simulink model "halate_koli"  (R2015a)
settings: Solver=ode45  StartTime=0.02  StopTime=0.04  RelTol=1e-3
libraries: powerlib x41, simulink x14, powerlib_meascontrol x14, dspstat3 x2
settings Model: Creator=yahya  LastModifiedBy=Yahya

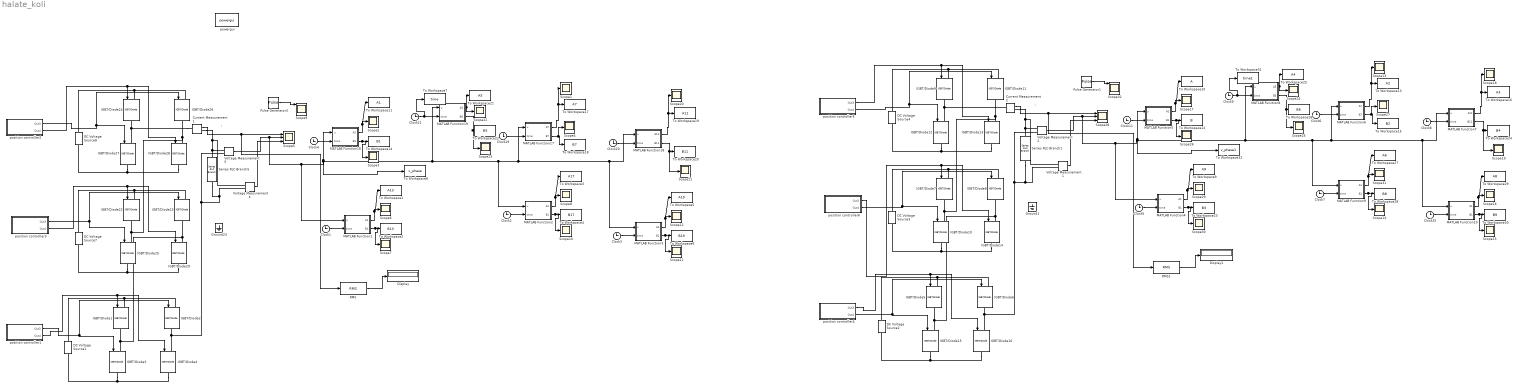
== system halate_koli ==
  note: i
  note: i
  Clock{1..11,19..21} (14 alike) : Clock
  Current Measurement1 : powerlib/Measurements/Current Measurement  PhasorSimulation=off  OutputType=Complex  PSBequivalent=0
  Current Measurement2 : powerlib/Measurements/Current Measurement  PhasorSimulation=off  OutputType=Complex  PSBequivalent=0
  DC Voltage Source{1..4,7..8} (6 alike) : powerlib/Electrical Sources/DC Voltage Source  Amplitude=100  Measurements=None
  Display : Display
  Display1 : Display
  Ground1 : powerlib/Elements/Ground  LConnTagsString=a
  Ground23 : powerlib/Elements/Ground  LConnTagsString=a
  IGBT/Diode{1..16,22..29} (24 alike) : powerlib/Power Electronics/IGBT//Diode  Ron=1e-3  Rs=1e5  Cs=inf  Measurements=off
  MATLAB Function1 : MATLAB Function  TreatAsAtomicUnit=on
  MATLAB Function10 : MATLAB Function  TreatAsAtomicUnit=on
  MATLAB Function16 : MATLAB Function  TreatAsAtomicUnit=on
  MATLAB Function17 : MATLAB Function  TreatAsAtomicUnit=on
  MATLAB Function18 : MATLAB Function  TreatAsAtomicUnit=on
  MATLAB Function19 : MATLAB Function  TreatAsAtomicUnit=on
  MATLAB Function2 : MATLAB Function  TreatAsAtomicUnit=on
  MATLAB Function3 : MATLAB Function  TreatAsAtomicUnit=on
  MATLAB Function4 : MATLAB Function  TreatAsAtomicUnit=on
  MATLAB Function5 : MATLAB Function  TreatAsAtomicUnit=on
  MATLAB Function6 : MATLAB Function  TreatAsAtomicUnit=on
  MATLAB Function7 : MATLAB Function  TreatAsAtomicUnit=on
  MATLAB Function8 : MATLAB Function  TreatAsAtomicUnit=on
  MATLAB Function9 : MATLAB Function  TreatAsAtomicUnit=on
  Pulse Generator1 : DiscretePulseGenerator  PulseType=Time based  Amplitude=0.8  Period=0.00001  PulseWidth=50
  Pulse Generator3 : DiscretePulseGenerator  PulseType=Time based  Amplitude=0.8  Period=0.00001  PulseWidth=50
  RMS : dspstat3/RMS  run=off  reset_popup=None  InputProcessing=Columns as channels (frame based)  directionMode=Each column  dimension=1  treatSBRowAsCol=off
  RMS1 : dspstat3/RMS  run=off  reset_popup=None  InputProcessing=Columns as channels (frame based)  directionMode=Each column  dimension=1  treatSBRowAsCol=off
  Scope{1..4,6..8,10..27,29..31} (28 alike) : Scope
      Scope1 settings: TimeRange=0.2  YMin=190  YMax=400  SaveName=ScopeData6
      Scope10 settings: TimeRange=0.2  YMin=190  YMax=400  SaveName=ScopeData12
      Scope11 settings: TimeRange=0.2  YMin=190  YMax=400  SaveName=ScopeData14
      Scope12 settings: TimeRange=0.2  YMin=190  YMax=400  SaveName=ScopeData24
      Scope13 settings: TimeRange=0.2  YMin=190  YMax=400  SaveName=ScopeData2
      Scope14 settings: TimeRange=0.2  YMin=190  YMax=400  SaveName=ScopeData4
      Scope15 settings: TimeRange=0.2  YMin=190  YMax=400  SaveName=ScopeData5
      Scope16 settings: TimeRange=0.2  YMin=190  YMax=400  SaveName=ScopeData8
      Scope17 settings: TimeRange=0.2  YMin=190  YMax=400  SaveName=ScopeData15
      Scope18 settings: TimeRange=0.2  YMin=190  YMax=400  SaveName=ScopeData16
      Scope19 settings: TimeRange=0.2  YMin=190  YMax=400  SaveName=ScopeData17
      Scope2 settings: TimeRange=0.2  YMin=190  YMax=400  SaveName=ScopeData7
      Scope20 settings: TimeRange=0.2  YMin=190  YMax=400  SaveName=ScopeData20
      Scope21 settings: TimeRange=0.2  YMin=190  YMax=400  SaveName=ScopeData21
      Scope22 settings: TimeRange=0.2  YMin=190  YMax=400  SaveName=ScopeData22
      Scope23 settings: TimeRange=0.2  YMin=190  YMax=400  SaveName=ScopeData23
      Scope24 settings: TimeRange=0.2  YMin=190  YMax=400  SaveName=ScopeData25
      Scope25 settings: TimeRange=0.2  YMin=190  YMax=400  SaveName=ScopeData26
      Scope26 settings: TimeRange=0.2  YMin=190  YMax=400  SaveName=ScopeData27
      Scope27 settings: TimeRange=0.2  YMin=190  YMax=400  SaveName=ScopeData28
      Scope29 settings: TimeRange=0.2  YMin=190  YMax=400  SaveName=ScopeData30
      Scope3 settings: TimeRange=0.2  YMin=190  YMax=400  SaveName=ScopeData9
      Scope30 settings: TimeRange=0.2  YMin=190  YMax=400  SaveName=ScopeData31
      Scope31 settings: TimeRange=0.2  YMin=190  YMax=400  SaveName=ScopeData32
      Scope4 settings: TimeRange=0.2  YMin=190  YMax=400  SaveName=ScopeData19
      Scope6 settings: TimeRange=0.2  YMin=190  YMax=400  SaveName=ScopeData10
      Scope7 settings: TimeRange=0.2  YMin=190  YMax=400  SaveName=ScopeData11
      Scope8 settings: TimeRange=0.2  YMin=190  YMax=400  SaveName=ScopeData13
  Scope28 : Scope  NumInputPorts=3
      settings: TimeRange=1  YMin=-400~-400~-5  YMax=400~400~5  SaveName=ScopeData29
  Scope32 : Scope  NumInputPorts=4
      settings: YMin=-5~-5~-5~-5  YMax=5~5~5~5  SaveName=ScopeData33
  Scope5 : Scope  NumInputPorts=3
      settings: TimeRange=1  YMin=-400~-400~-5  YMax=400~400~5  SaveName=ScopeData3
  Scope9 : Scope  NumInputPorts=4
      settings: YMin=-5~-5~-5~-5  YMax=5~5~5~5  SaveName=ScopeData18
  Series RLC Branch1 : powerlib/Elements/Series RLC Branch  LConnTagsString=__new0  RConnTagsString=__new0  BranchType=R  Resistance=330  Inductance=1e-5  SetiL0=off  InitialCurrent=0  Capacitance=1e-6  Setx0=off  InitialVoltage=0  Measurements=None
  Series RLC Branch5 : powerlib/Elements/Series RLC Branch  LConnTagsString=__new0  RConnTagsString=__new0  BranchType=R  Resistance=1  Inductance=1e-5  SetiL0=off  InitialCurrent=0  Capacitance=1e-6  Setx0=off  InitialVoltage=0  Measurements=None
  To Workspace1 : ToWorkspace  VariableName=A13  SaveFormat=Timeseries  SampleTime=-1
  To Workspace10 : ToWorkspace  VariableName=A  SaveFormat=Timeseries  SampleTime=-1
  To Workspace11 : ToWorkspace  VariableName=A1  SaveFormat=Timeseries  SampleTime=-1
  To Workspace12 : ToWorkspace  VariableName=B  SaveFormat=Timeseries  SampleTime=-1
  To Workspace13 : ToWorkspace  VariableName=A2  SaveFormat=Timeseries  SampleTime=-1
  To Workspace14 : ToWorkspace  VariableName=B1  SaveFormat=Timeseries  SampleTime=-1
  To Workspace15 : ToWorkspace  VariableName=B2  SaveFormat=Timeseries  SampleTime=-1
  To Workspace16 : ToWorkspace  VariableName=A3  SaveFormat=Timeseries  SampleTime=-1
  To Workspace17 : ToWorkspace  VariableName=A7  SaveFormat=Timeseries  SampleTime=-1
  To Workspace18 : ToWorkspace  VariableName=B7  SaveFormat=Timeseries  SampleTime=-1
  To Workspace19 : ToWorkspace  VariableName=A11  SaveFormat=Timeseries  SampleTime=-1
  To Workspace2 : ToWorkspace  VariableName=B13  SaveFormat=Timeseries  SampleTime=-1
  To Workspace20 : ToWorkspace  VariableName=B11  SaveFormat=Timeseries  SampleTime=-1
  To Workspace21 : ToWorkspace  VariableName=A5  SaveFormat=Timeseries  SampleTime=-1
  To Workspace22 : ToWorkspace  VariableName=B5  SaveFormat=Timeseries  SampleTime=-1
  To Workspace23 : ToWorkspace  VariableName=B3  SaveFormat=Timeseries  SampleTime=-1
  To Workspace24 : ToWorkspace  VariableName=B4  SaveFormat=Timeseries  SampleTime=-1
  To Workspace25 : ToWorkspace  VariableName=A4  SaveFormat=Timeseries  SampleTime=-1
  To Workspace26 : ToWorkspace  VariableName=B6  SaveFormat=Timeseries  SampleTime=-1
  To Workspace27 : ToWorkspace  VariableName=A6  SaveFormat=Timeseries  SampleTime=-1
  To Workspace28 : ToWorkspace  VariableName=B8  SaveFormat=Timeseries  SampleTime=-1
  To Workspace29 : ToWorkspace  VariableName=A8  SaveFormat=Timeseries  SampleTime=-1
  To Workspace3 : ToWorkspace  VariableName=A17  SaveFormat=Timeseries  SampleTime=-1
  To Workspace30 : ToWorkspace  VariableName=B9  SaveFormat=Timeseries  SampleTime=-1
  To Workspace31 : ToWorkspace  VariableName=time1  SaveFormat=Timeseries  SampleTime=-1
  To Workspace32 : ToWorkspace  VariableName=v_phase1  SaveFormat=Timeseries  SampleTime=-1
  To Workspace4 : ToWorkspace  VariableName=B17  SaveFormat=Timeseries  SampleTime=-1
  To Workspace5 : ToWorkspace  VariableName=A19  SaveFormat=Timeseries  SampleTime=-1
  To Workspace6 : ToWorkspace  VariableName=B19  SaveFormat=Timeseries  SampleTime=-1
  To Workspace7 : ToWorkspace  VariableName=time  SaveFormat=Timeseries  SampleTime=-1
  To Workspace8 : ToWorkspace  VariableName=v_phase  SaveFormat=Timeseries  SampleTime=-1
  To Workspace9 : ToWorkspace  VariableName=A9  SaveFormat=Timeseries  SampleTime=-1
  Voltage Measurement{1..2,4..5} (4 alike) : powerlib/Measurements/Voltage Measurement  PhasorSimulation=off  OutputType=Complex  PSBequivalent=0
  position controller1 : Subsystem
  position controller2 : Subsystem
  position controller3 : Subsystem
  position controller4 : Subsystem
  position controller5 : Subsystem
  position controller6 : Subsystem
  powergui : powerlib/powergui  Priority=1  SimulationMode=Continuous  SolverType=Tustin/Backward Euler (TBE)  SampleTime=50e-6  frequency=60  SPID=off  DisableSnubberDevices=off  DisableRonSwitches=off  DisableVfSwitches=off  SwTol=0  DisplayEquations=off  Interpol=off  methode=off  Ts=100  FunctionMessages=off  echomessages=off  HookPort=off  EnableUseOfTLC=off  x0status=blocks  frequencyindice=0  Pbase=100e6  ErrMax=1e-4  Iterations=50  UnitsV=kV  UnitsW=MW  buscounter=0  RestoreLinks=warning  ResistiveCurrentMeasurement=off  Frange=[0:2:500]  Ylog=off  Xlog=on  ShowGrid=off  save=off  variable=ZData  structure=0  ZoomFFT=off  StartTime=0.0  cycles=1  DisplayStyle=1  fundamental=60  FreqAxis=off  MaxFrequency=1000  frequencyindicesteady=1  RmsSteady=1  display=off
  wires:
  position controller2/2(Out4) -> IGBT/Diode28/1, IGBT/Diode24/1
  position controller2/1(Out3) -> IGBT/Diode26/1, IGBT/Diode27/1
  position controller3/2(Out4) -> IGBT/Diode29/1, IGBT/Diode22/1
  position controller3/1(Out3) -> IGBT/Diode23/1, IGBT/Diode25/1
  Voltage Measurement4/1 -> Scope5/3
  position controller1/2(Out4) -> IGBT/Diode4/1, IGBT/Diode1/1
  position controller1/1(Out3) -> IGBT/Diode3/1, IGBT/Diode2/1
  Clock4/1 -> MATLAB Function16/2(time)
  MATLAB Function16/1(A1) -> To Workspace11/1, Scope2/1
  MATLAB Function16/2(B1) -> Scope3/1, To Workspace14/1
  Clock19/1 -> MATLAB Function17/2(time)
  MATLAB Function17/1(A7) -> Scope1/1, To Workspace17/1
  MATLAB Function17/2(B7) -> To Workspace18/1, Scope4/1
  Clock20/1 -> MATLAB Function18/2(time)
  MATLAB Function18/1(A11) -> Scope20/1, To Workspace19/1
  MATLAB Function18/2(B11) -> Scope21/1, To Workspace20/1
  MATLAB Function19/1(A5) -> Scope22/1, To Workspace21/1
  MATLAB Function19/2(B5) -> Scope23/1, To Workspace22/1
  Clock1/1 -> MATLAB Function1/2(time)
  MATLAB Function1/1(A1) -> To Workspace1/1, Scope6/1
  MATLAB Function1/2(B1) -> Scope7/1, To Workspace2/1
  Clock2/1 -> MATLAB Function2/2(time)
  MATLAB Function2/1(A1) -> To Workspace3/1, Scope8/1
  MATLAB Function2/2(B1) -> Scope10/1, To Workspace4/1
  Clock3/1 -> MATLAB Function3/2(time)
  MATLAB Function3/1(A1) -> To Workspace5/1, Scope12/1
  MATLAB Function3/2(B1) -> Scope11/1, To Workspace6/1
  Voltage Measurement5/1 -> MATLAB Function1/1(u), MATLAB Function2/1(u), MATLAB Function3/1(u), MATLAB Function18/1(u), MATLAB Function17/1(u), MATLAB Function19/1(u), To Workspace8/1, MATLAB Function16/1(u), Scope5/2
  Clock21/1 -> To Workspace7/1, MATLAB Function19/2(time)
  Pulse Generator3/1 -> Scope9/1
  Current Measurement1/1 -> RMS/1, Scope5/1
  RMS/1 -> Display/1
  position controller5/1(Out3) -> IGBT/Diode13/1, IGBT/Diode9/1
  position controller5/2(Out4) -> IGBT/Diode11/1, IGBT/Diode12/1
  position controller6/1(Out3) -> IGBT/Diode14/1, IGBT/Diode7/1
  position controller6/2(Out4) -> IGBT/Diode8/1, IGBT/Diode10/1
  Voltage Measurement1/1 -> Scope28/3
  position controller4/1(Out3) -> IGBT/Diode16/1, IGBT/Diode5/1
  position controller4/2(Out4) -> IGBT/Diode15/1, IGBT/Diode6/1
  Clock11/1 -> MATLAB Function5/2(time)
  MATLAB Function5/1(A1) -> To Workspace10/1, Scope17/1
  MATLAB Function5/2(B1) -> Scope26/1, To Workspace12/1
  Clock6/1 -> MATLAB Function6/2(time)
  MATLAB Function6/1(A7) -> Scope13/1, To Workspace13/1
  MATLAB Function6/2(B7) -> To Workspace15/1, Scope27/1
  Clock8/1 -> MATLAB Function7/2(time)
  MATLAB Function7/1(A11) -> Scope18/1, To Workspace16/1
  MATLAB Function7/2(B11) -> Scope19/1, To Workspace24/1
  MATLAB Function8/1(A5) -> Scope24/1, To Workspace25/1
  MATLAB Function8/2(B5) -> Scope25/1, To Workspace26/1
  Clock5/1 -> MATLAB Function4/2(time)
  MATLAB Function4/1(A1) -> To Workspace9/1, Scope29/1
  MATLAB Function4/2(B1) -> Scope30/1, To Workspace23/1
  Clock7/1 -> MATLAB Function9/2(time)
  MATLAB Function9/1(A1) -> To Workspace27/1, Scope31/1
  MATLAB Function9/2(B1) -> Scope14/1, To Workspace28/1
  Clock10/1 -> MATLAB Function10/2(time)
  MATLAB Function10/1(A1) -> To Workspace29/1, Scope16/1
  MATLAB Function10/2(B1) -> Scope15/1, To Workspace30/1
  Voltage Measurement2/1 -> MATLAB Function4/1(u), MATLAB Function9/1(u), MATLAB Function10/1(u), MATLAB Function7/1(u), MATLAB Function6/1(u), MATLAB Function8/1(u), To Workspace32/1, MATLAB Function5/1(u), Scope28/2
  Clock9/1 -> To Workspace31/1, MATLAB Function8/2(time)
  Pulse Generator1/1 -> Scope32/1
  Current Measurement2/1 -> RMS1/1, Scope28/1
  RMS1/1 -> Display1/1
  connections:
  IGBT/Diode24/LConn1 -- DC Voltage Source8/RConn1 -- IGBT/Diode26/LConn1
  IGBT/Diode28/RConn1 -- DC Voltage Source8/LConn1 -- IGBT/Diode27/RConn1
  Current Measurement1/LConn1 -- IGBT/Diode24/RConn1 -- IGBT/Diode27/LConn1
  IGBT/Diode22/LConn1 -- DC Voltage Source7/RConn1 -- IGBT/Diode23/LConn1
  IGBT/Diode25/RConn1 -- DC Voltage Source7/LConn1 -- IGBT/Diode29/RConn1
  IGBT/Diode26/RConn1 -- IGBT/Diode28/LConn1 -- IGBT/Diode22/RConn1 -- IGBT/Diode25/LConn1
  IGBT/Diode1/RConn1 -- IGBT/Diode3/LConn1 -- IGBT/Diode29/LConn1 -- IGBT/Diode23/RConn1
  Current Measurement1/RConn1 -- Voltage Measurement4/LConn1 -- Voltage Measurement5/LConn1 -- Series RLC Branch5/LConn1
  IGBT/Diode2/LConn1 -- IGBT/Diode1/LConn1 -- DC Voltage Source1/RConn1
  IGBT/Diode4/RConn1 -- IGBT/Diode3/RConn1 -- DC Voltage Source1/LConn1
  IGBT/Diode2/RConn1 -- Series RLC Branch5/RConn1 -- Voltage Measurement4/LConn2 -- Voltage Measurement5/LConn2 -- IGBT/Diode4/LConn1
  IGBT/Diode11/LConn1 -- IGBT/Diode9/LConn1 -- DC Voltage Source4/RConn1
  IGBT/Diode12/RConn1 -- IGBT/Diode13/RConn1 -- DC Voltage Source4/LConn1
  IGBT/Diode12/LConn1 -- Current Measurement2/LConn1 -- IGBT/Diode9/RConn1
  IGBT/Diode8/LConn1 -- IGBT/Diode7/LConn1 -- DC Voltage Source3/RConn1
  IGBT/Diode14/RConn1 -- IGBT/Diode10/RConn1 -- DC Voltage Source3/LConn1
  IGBT/Diode10/LConn1 -- IGBT/Diode7/RConn1 -- IGBT/Diode11/RConn1 -- IGBT/Diode13/LConn1
  IGBT/Diode8/RConn1 -- IGBT/Diode14/LConn1 -- IGBT/Diode5/RConn1 -- IGBT/Diode15/LConn1
  Series RLC Branch1/LConn1 -- Voltage Measurement2/LConn1 -- Current Measurement2/RConn1 -- Voltage Measurement1/LConn1
  DC Voltage Source2/RConn1 -- IGBT/Diode6/LConn1 -- IGBT/Diode5/LConn1
  DC Voltage Source2/LConn1 -- IGBT/Diode16/RConn1 -- IGBT/Diode15/RConn1
  IGBT/Diode16/LConn1 -- Series RLC Branch1/RConn1 -- Voltage Measurement1/LConn2 -- Voltage Measurement2/LConn2 -- IGBT/Diode6/RConn1

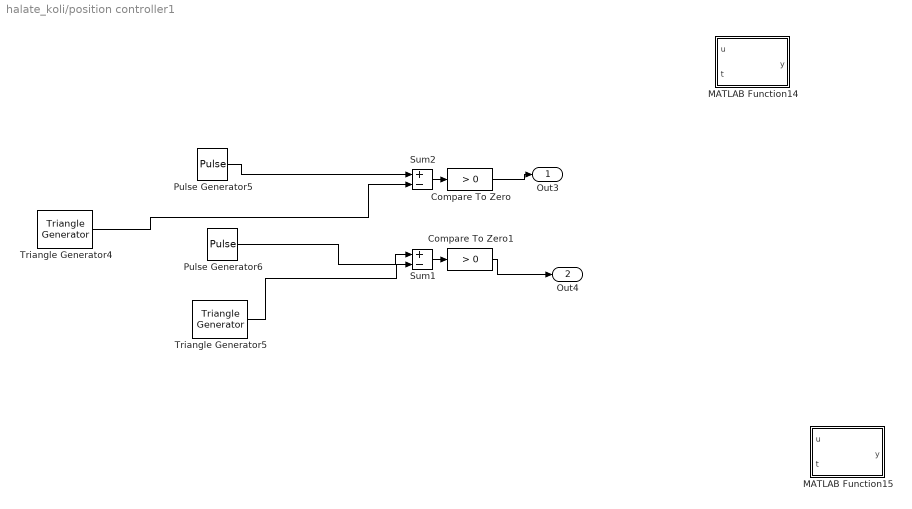
== system halate_koli/position controller1 ==
  Compare To Zero : simulink/Logic and Bit Operations/Compare To Zero  relop=>  OutDataTypeStr=boolean  ZeroCross=off
  Compare To Zero1 : simulink/Logic and Bit Operations/Compare To Zero  relop=>  OutDataTypeStr=boolean  ZeroCross=off
  MATLAB Function14 : MATLAB Function  TreatAsAtomicUnit=on
  MATLAB Function15 : MATLAB Function  TreatAsAtomicUnit=on
  Pulse Generator5 : DiscretePulseGenerator  PulseType=Time based  Amplitude=0.1254  Period=0.02  PulseWidth=50.001
  Pulse Generator6 : DiscretePulseGenerator  PulseType=Time based  Amplitude=0.1254  Period=0.02  PulseWidth=50.001  PhaseDelay=0.01
  Sum1 : Sum  Inputs=+-  OutDataTypeStr=double
  Sum2 : Sum  Inputs=+-  OutDataTypeStr=double
  Triangle Generator4 : powerlib_meascontrol/Pulse & Signal Generators/Triangle Generator  Freq=50  Phase=90  Ts=0
  Triangle Generator5 : powerlib_meascontrol/Pulse & Signal Generators/Triangle Generator  Freq=50  Phase=90+180  Ts=0
  Out3 : Outport
  Out4 : Outport  Port=2
  wires:
  Compare To Zero/1 -> Out3/1
  Compare To Zero1/1 -> Out4/1
  Triangle Generator4/1 -> Sum2/2
  Sum2/1 -> Compare To Zero/1
  Sum1/1 -> Compare To Zero1/1
  Pulse Generator5/1 -> Sum2/1
  Pulse Generator6/1 -> Sum1/1
  Triangle Generator5/1 -> Sum1/2

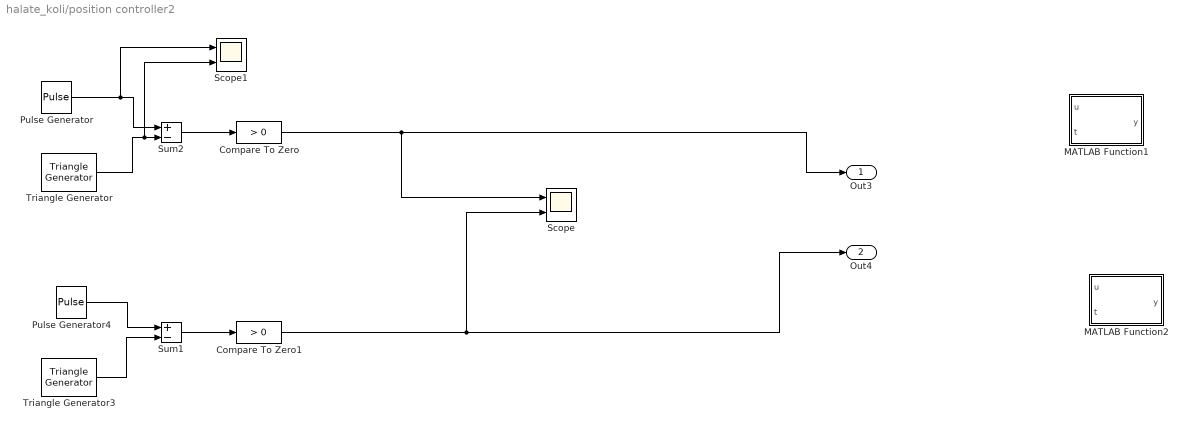
== system halate_koli/position controller2 ==
  Compare To Zero : simulink/Logic and Bit Operations/Compare To Zero  relop=>  OutDataTypeStr=boolean  ZeroCross=off
  Compare To Zero1 : simulink/Logic and Bit Operations/Compare To Zero  relop=>  OutDataTypeStr=boolean  ZeroCross=off
  MATLAB Function1 : MATLAB Function  TreatAsAtomicUnit=on
  MATLAB Function2 : MATLAB Function  TreatAsAtomicUnit=on
  Pulse Generator : DiscretePulseGenerator  PulseType=Time based  Amplitude=0.6526  Period=0.02  PulseWidth=50.001
  Pulse Generator4 : DiscretePulseGenerator  PulseType=Time based  Amplitude=0.6526  Period=0.02  PulseWidth=50.001  PhaseDelay=0.01
  Scope : Scope  NumInputPorts=2
      settings: YMin=-5~-5  YMax=5~5
  Scope1 : Scope  NumInputPorts=2
      settings: YMin=-5~-5  YMax=5~5
  Sum1 : Sum  Inputs=+-  OutDataTypeStr=double
  Sum2 : Sum  Inputs=+-  OutDataTypeStr=double
  Triangle Generator : powerlib_meascontrol/Pulse & Signal Generators/Triangle Generator  Freq=50  Phase=90  Ts=0
  Triangle Generator3 : powerlib_meascontrol/Pulse & Signal Generators/Triangle Generator  Freq=50  Phase=90+180  Ts=0
  Out3 : Outport
  Out4 : Outport  Port=2
  wires:
  Pulse Generator/1 -> Scope1/1, Sum2/1
  Triangle Generator/1 -> Scope1/2, Sum2/2
  Pulse Generator4/1 -> Sum1/1
  Triangle Generator3/1 -> Sum1/2
  Compare To Zero1/1 -> Scope/2, Out4/1
  Sum2/1 -> Compare To Zero/1
  Sum1/1 -> Compare To Zero1/1
  Compare To Zero/1 -> Scope/1, Out3/1

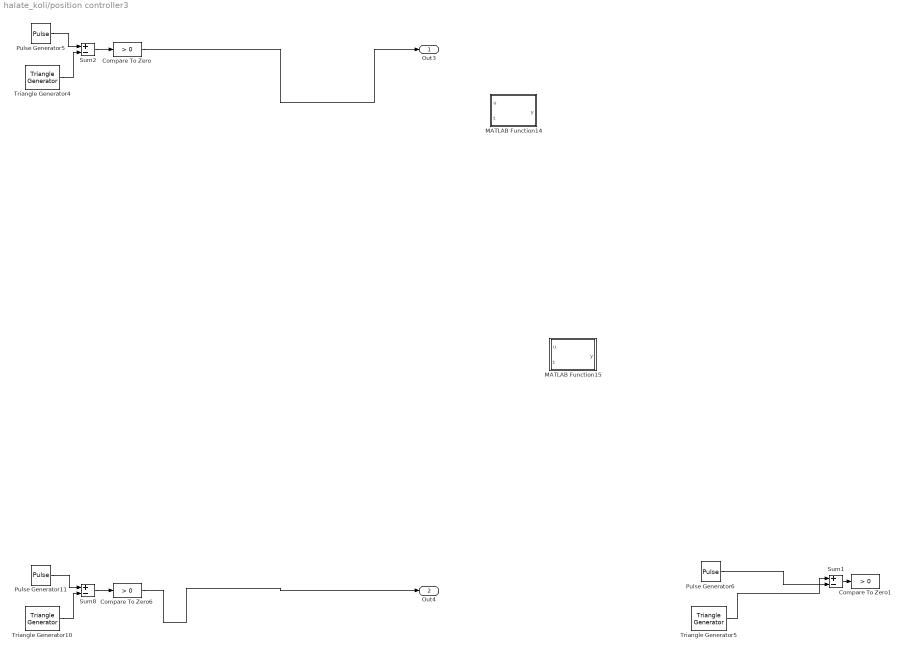
== system halate_koli/position controller3 ==
  Compare To Zero : simulink/Logic and Bit Operations/Compare To Zero  relop=>  OutDataTypeStr=boolean  ZeroCross=off
  Compare To Zero1 : simulink/Logic and Bit Operations/Compare To Zero  relop=>  OutDataTypeStr=boolean  ZeroCross=off
  Compare To Zero6 : simulink/Logic and Bit Operations/Compare To Zero  relop=>  OutDataTypeStr=boolean  ZeroCross=off
  MATLAB Function14 : MATLAB Function  TreatAsAtomicUnit=on
  MATLAB Function15 : MATLAB Function  TreatAsAtomicUnit=on
  Pulse Generator11 : DiscretePulseGenerator  PulseType=Time based  Amplitude=0.3487  Period=0.02  PulseWidth=50.001  PhaseDelay=0.01
  Pulse Generator5 : DiscretePulseGenerator  PulseType=Time based  Amplitude=0.3487  Period=0.02  PulseWidth=50.001
  Pulse Generator6 : DiscretePulseGenerator  PulseType=Time based  Amplitude=0.332  Period=0.02  PulseWidth=50  PhaseDelay=0.01
  Sum1 : Sum  Inputs=+-  OutDataTypeStr=double
  Sum2 : Sum  Inputs=+-  OutDataTypeStr=double
  Sum8 : Sum  Inputs=+-  OutDataTypeStr=double
  Triangle Generator10 : powerlib_meascontrol/Pulse & Signal Generators/Triangle Generator  Freq=50  Phase=90+180  Ts=0
  Triangle Generator4 : powerlib_meascontrol/Pulse & Signal Generators/Triangle Generator  Freq=50  Phase=90  Ts=0
  Triangle Generator5 : powerlib_meascontrol/Pulse & Signal Generators/Triangle Generator  Freq=50  Phase=90+180  Ts=0
  Out3 : Outport
  Out4 : Outport  Port=2
  wires:
  Triangle Generator4/1 -> Sum2/2
  Sum2/1 -> Compare To Zero/1
  Sum1/1 -> Compare To Zero1/1
  Pulse Generator5/1 -> Sum2/1
  Pulse Generator6/1 -> Sum1/1
  Triangle Generator5/1 -> Sum1/2
  Compare To Zero/1 -> Out3/1
  Triangle Generator10/1 -> Sum8/2
  Sum8/1 -> Compare To Zero6/1
  Pulse Generator11/1 -> Sum8/1
  Compare To Zero6/1 -> Out4/1

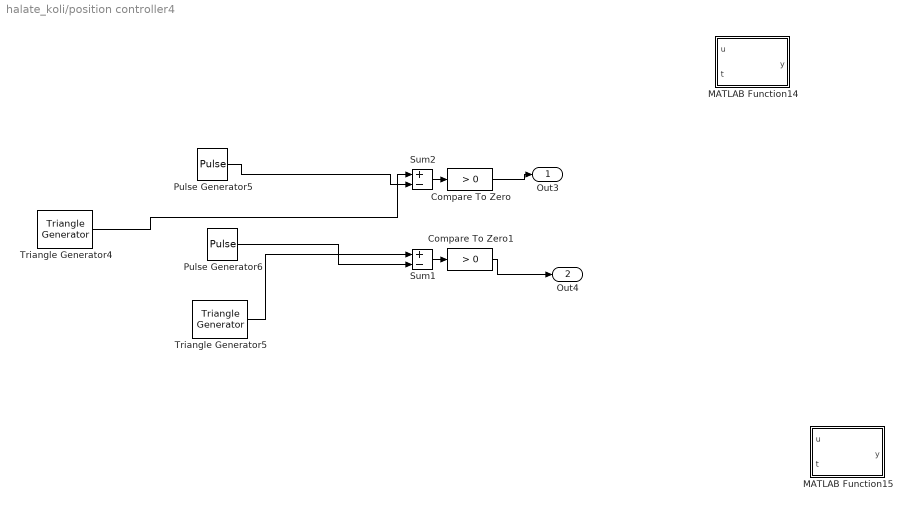
== system halate_koli/position controller4 ==
  Compare To Zero : simulink/Logic and Bit Operations/Compare To Zero  relop=>  OutDataTypeStr=boolean  ZeroCross=off
  Compare To Zero1 : simulink/Logic and Bit Operations/Compare To Zero  relop=>  OutDataTypeStr=boolean  ZeroCross=off
  MATLAB Function14 : MATLAB Function  TreatAsAtomicUnit=on
  MATLAB Function15 : MATLAB Function  TreatAsAtomicUnit=on
  Pulse Generator5 : DiscretePulseGenerator  PulseType=Time based  Amplitude=0.1254  Period=0.02  PulseWidth=50.001
  Pulse Generator6 : DiscretePulseGenerator  PulseType=Time based  Amplitude=0.1254  Period=0.02  PulseWidth=50.001  PhaseDelay=0.01
  Sum1 : Sum  Inputs=+-  OutDataTypeStr=double
  Sum2 : Sum  Inputs=+-  OutDataTypeStr=double
  Triangle Generator4 : powerlib_meascontrol/Pulse & Signal Generators/Triangle Generator  Freq=50  Phase=90  Ts=0
  Triangle Generator5 : powerlib_meascontrol/Pulse & Signal Generators/Triangle Generator  Freq=50  Phase=90+180  Ts=0
  Out3 : Outport
  Out4 : Outport  Port=2
  wires:
  Compare To Zero/1 -> Out3/1
  Compare To Zero1/1 -> Out4/1
  Triangle Generator4/1 -> Sum2/1
  Sum2/1 -> Compare To Zero/1
  Sum1/1 -> Compare To Zero1/1
  Pulse Generator5/1 -> Sum2/2
  Pulse Generator6/1 -> Sum1/2
  Triangle Generator5/1 -> Sum1/1

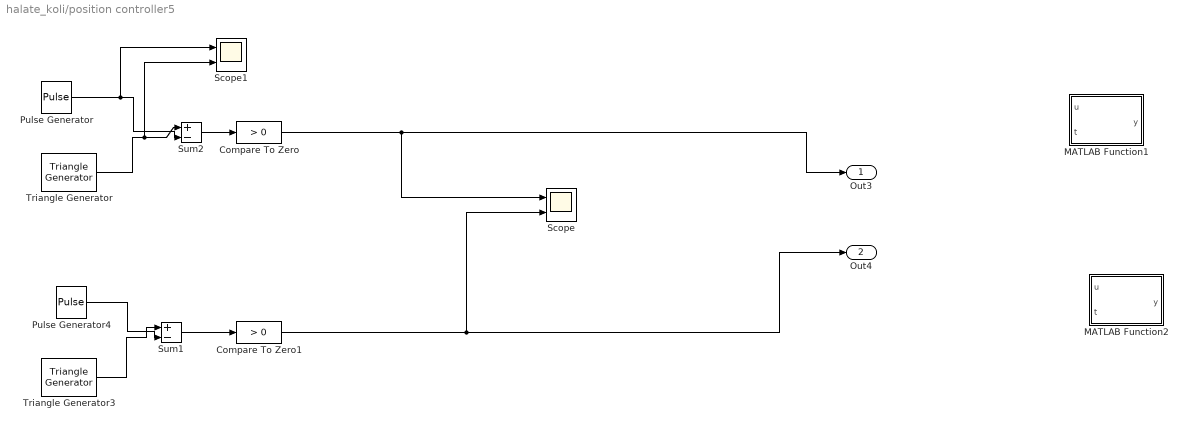
== system halate_koli/position controller5 ==
  Compare To Zero : simulink/Logic and Bit Operations/Compare To Zero  relop=>  OutDataTypeStr=boolean  ZeroCross=off
  Compare To Zero1 : simulink/Logic and Bit Operations/Compare To Zero  relop=>  OutDataTypeStr=boolean  ZeroCross=off
  MATLAB Function1 : MATLAB Function  TreatAsAtomicUnit=on
  MATLAB Function2 : MATLAB Function  TreatAsAtomicUnit=on
  Pulse Generator : DiscretePulseGenerator  PulseType=Time based  Amplitude=0.6526  Period=0.02  PulseWidth=50.001
  Pulse Generator4 : DiscretePulseGenerator  PulseType=Time based  Amplitude=0.6526  Period=0.02  PulseWidth=50.001  PhaseDelay=0.01
  Scope : Scope  NumInputPorts=2
      settings: YMin=-5~-5  YMax=5~5
  Scope1 : Scope  NumInputPorts=2
      settings: YMin=-5~-5  YMax=5~5
  Sum1 : Sum  Inputs=+-  OutDataTypeStr=double
  Sum2 : Sum  Inputs=+-  OutDataTypeStr=double
  Triangle Generator : powerlib_meascontrol/Pulse & Signal Generators/Triangle Generator  Freq=50  Phase=90  Ts=0
  Triangle Generator3 : powerlib_meascontrol/Pulse & Signal Generators/Triangle Generator  Freq=50  Phase=90+180  Ts=0
  Out3 : Outport
  Out4 : Outport  Port=2
  wires:
  Pulse Generator/1 -> Sum2/2, Scope1/1
  Triangle Generator/1 -> Sum2/1, Scope1/2
  Pulse Generator4/1 -> Sum1/2
  Triangle Generator3/1 -> Sum1/1
  Compare To Zero1/1 -> Scope/2, Out4/1
  Sum2/1 -> Compare To Zero/1
  Sum1/1 -> Compare To Zero1/1
  Compare To Zero/1 -> Scope/1, Out3/1

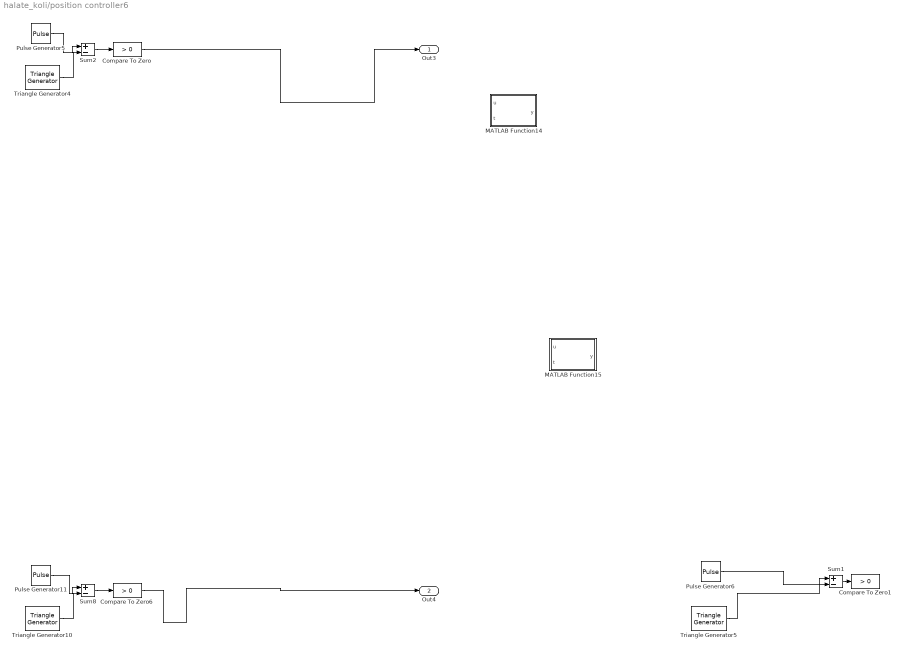
== system halate_koli/position controller6 ==
  Compare To Zero : simulink/Logic and Bit Operations/Compare To Zero  relop=>  OutDataTypeStr=boolean  ZeroCross=off
  Compare To Zero1 : simulink/Logic and Bit Operations/Compare To Zero  relop=>  OutDataTypeStr=boolean  ZeroCross=off
  Compare To Zero6 : simulink/Logic and Bit Operations/Compare To Zero  relop=>  OutDataTypeStr=boolean  ZeroCross=off
  MATLAB Function14 : MATLAB Function  TreatAsAtomicUnit=on
  MATLAB Function15 : MATLAB Function  TreatAsAtomicUnit=on
  Pulse Generator11 : DiscretePulseGenerator  PulseType=Time based  Amplitude=0.3487  Period=0.02  PulseWidth=50.001  PhaseDelay=0.01
  Pulse Generator5 : DiscretePulseGenerator  PulseType=Time based  Amplitude=0.3487  Period=0.02  PulseWidth=50.001
  Pulse Generator6 : DiscretePulseGenerator  PulseType=Time based  Amplitude=0.332  Period=0.02  PulseWidth=50  PhaseDelay=0.01
  Sum1 : Sum  Inputs=+-  OutDataTypeStr=double
  Sum2 : Sum  Inputs=+-  OutDataTypeStr=double
  Sum8 : Sum  Inputs=+-  OutDataTypeStr=double
  Triangle Generator10 : powerlib_meascontrol/Pulse & Signal Generators/Triangle Generator  Freq=50  Phase=90+180  Ts=0
  Triangle Generator4 : powerlib_meascontrol/Pulse & Signal Generators/Triangle Generator  Freq=50  Phase=90  Ts=0
  Triangle Generator5 : powerlib_meascontrol/Pulse & Signal Generators/Triangle Generator  Freq=50  Phase=90+180  Ts=0
  Out3 : Outport
  Out4 : Outport  Port=2
  wires:
  Triangle Generator4/1 -> Sum2/1
  Sum2/1 -> Compare To Zero/1
  Sum1/1 -> Compare To Zero1/1
  Pulse Generator5/1 -> Sum2/2
  Pulse Generator6/1 -> Sum1/1
  Triangle Generator5/1 -> Sum1/2
  Compare To Zero/1 -> Out3/1
  Triangle Generator10/1 -> Sum8/1
  Sum8/1 -> Compare To Zero6/1
  Pulse Generator11/1 -> Sum8/2
  Compare To Zero6/1 -> Out4/1

== matlab function halate_koli/position controller3/MATLAB Function14 ==
  data: u input; y output; t input
function y = fcn(u,t)
%#codegen
if t>u
    y = 1;
else
    y = 0;
end
end

== matlab function halate_koli/MATLAB Function10 ==
  data: u input; A1 output; time input; B1 output
function [A1,B1] = fcn(u,time)
%#codegen
A1 = u*sin(19*2*pi*50*time);
B1 = u*cos(19*2*pi*50*time);
end

== matlab function halate_koli/position controller1/MATLAB Function14 ==
  data: u input; y output; t input
function y = fcn(u,t)
%#codegen
if t>u
    y = 1;
else
    y = 0;
end
end

== matlab function halate_koli/MATLAB Function4 ==
  data: u input; A1 output; time input; B1 output
function [A1,B1] = fcn(u,time)
%#codegen
A1 = u*sin(13*2*pi*50*time);
B1 = u*cos(13*2*pi*50*time);
end

== matlab function halate_koli/position controller2/MATLAB Function1 ==
  data: u input; y output; t input
function y = fcn(u,t)
%#codegen
if t>u
    y = 1;
else
    y = 0;
end
end

== matlab function halate_koli/position controller2/MATLAB Function2 ==
  data: u input; y output; t input
function y = fcn(u,t)
%#codegen
if t>u
    y = 1;
else
    y = 0;
end
end

== matlab function halate_koli/position controller1/MATLAB Function15 ==
  data: u input; y output; t input
function y = fcn(u,t)
%#codegen
if t>u
    y = 1;
else
    y = 0;
end
end

== matlab function halate_koli/MATLAB Function18 ==
  data: u input; A11 output; time input; B11 output
function [A11,B11] = fcn(u,time)
%#codegen
A11 = u*sin(11*2*pi*50*time);
B11 = u*cos(11*2*pi*50*time);
end

== matlab function halate_koli/MATLAB Function19 ==
  data: u input; A5 output; time input; B5 output
function [A5,B5] = fcn(u,time)
%#codegen
A5 = u*sin(5*2*pi*50*time);
B5 = u*cos(5*2*pi*50*time);
end

== matlab function halate_koli/MATLAB Function1 ==
  data: u input; A1 output; time input; B1 output
function [A1,B1] = fcn(u,time)
%#codegen
A1 = u*sin(13*2*pi*50*time);
B1 = u*cos(13*2*pi*50*time);
end

== matlab function halate_koli/MATLAB Function5 ==
  data: u input; A1 output; time input; B1 output
function [A1,B1] = fcn(u,time)
%#codegen
A1 = u*sin(2*pi*50*time);
B1 = u*cos(2*pi*50*time);
end

== matlab function halate_koli/MATLAB Function6 ==
  data: u input; A7 output; time input; B7 output
function [A7,B7] = fcn(u,time)
%#codegen
A7 = u*sin(7*2*pi*50*time);
B7 = u*cos(7*2*pi*50*time);
end

== matlab function halate_koli/MATLAB Function2 ==
  data: u input; A1 output; time input; B1 output
function [A1,B1] = fcn(u,time)
%#codegen
A1 = u*sin(17*2*pi*50*time);
B1 = u*cos(17*2*pi*50*time);
end

== matlab function halate_koli/MATLAB Function3 ==
  data: u input; A1 output; time input; B1 output
function [A1,B1] = fcn(u,time)
%#codegen
A1 = u*sin(19*2*pi*50*time);
B1 = u*cos(19*2*pi*50*time);
end

== matlab function halate_koli/MATLAB Function7 ==
  data: u input; A11 output; time input; B11 output
function [A11,B11] = fcn(u,time)
%#codegen
A11 = u*sin(11*2*pi*50*time);
B11 = u*cos(11*2*pi*50*time);
end

== matlab function halate_koli/position controller3/MATLAB Function15 ==
  data: u input; y output; t input
function y = fcn(u,t)
%#codegen
if t>u
    y = 1;
else
    y = 0;
end
end

== matlab function halate_koli/MATLAB Function16 ==
  data: u input; A1 output; time input; B1 output
function [A1,B1] = fcn(u,time)
%#codegen
A1 = u*sin(2*pi*50*time);
B1 = u*cos(2*pi*50*time);
end

== matlab function halate_koli/MATLAB Function17 ==
  data: u input; A7 output; time input; B7 output
function [A7,B7] = fcn(u,time)
%#codegen
A7 = u*sin(7*2*pi*50*time);
B7 = u*cos(7*2*pi*50*time);
end

== matlab function halate_koli/MATLAB Function8 ==
  data: u input; A5 output; time input; B5 output
function [A5,B5] = fcn(u,time)
%#codegen
A5 = u*sin(5*2*pi*50*time);
B5 = u*cos(5*2*pi*50*time);
end

== matlab function halate_koli/MATLAB Function9 ==
  data: u input; A1 output; time input; B1 output
function [A1,B1] = fcn(u,time)
%#codegen
A1 = u*sin(17*2*pi*50*time);
B1 = u*cos(17*2*pi*50*time);
end

== matlab function halate_koli/position controller4/MATLAB Function14 ==
  data: u input; y output; t input
function y = fcn(u,t)
%#codegen
if t>u
    y = 1;
else
    y = 0;
end
end

== matlab function halate_koli/position controller4/MATLAB Function15 ==
  data: u input; y output; t input
function y = fcn(u,t)
%#codegen
if t>u
    y = 1;
else
    y = 0;
end
end

== matlab function halate_koli/position controller5/MATLAB Function1 ==
  data: u input; y output; t input
function y = fcn(u,t)
%#codegen
if t>u
    y = 1;
else
    y = 0;
end
end

== matlab function halate_koli/position controller5/MATLAB Function2 ==
  data: u input; y output; t input
function y = fcn(u,t)
%#codegen
if t>u
    y = 1;
else
    y = 0;
end
end

== matlab function halate_koli/position controller6/MATLAB Function14 ==
  data: u input; y output; t input
function y = fcn(u,t)
%#codegen
if t>u
    y = 1;
else
    y = 0;
end
end

== matlab function halate_koli/position controller6/MATLAB Function15 ==
  data: u input; y output; t input
function y = fcn(u,t)
%#codegen
if t>u
    y = 1;
else
    y = 0;
end
end
